simulink model "tcs_VHF_PI_1"  (R2021a)
settings: Solver=FixedStepAuto  StartTime=0.0  StopTime=5  RelTol=1e-3
PreLoadFcn:
  | run('control_bus.m')
model workspace (MAT data in the model file):
  Tmax = 1000
libraries: simulink x2, Solver_SF x1
CloseFcn:
  | clear control_info_bus
settings Model: OrderedModelArguments=off  Creator=henri  LastModifiedBy=Henrique Mesquita

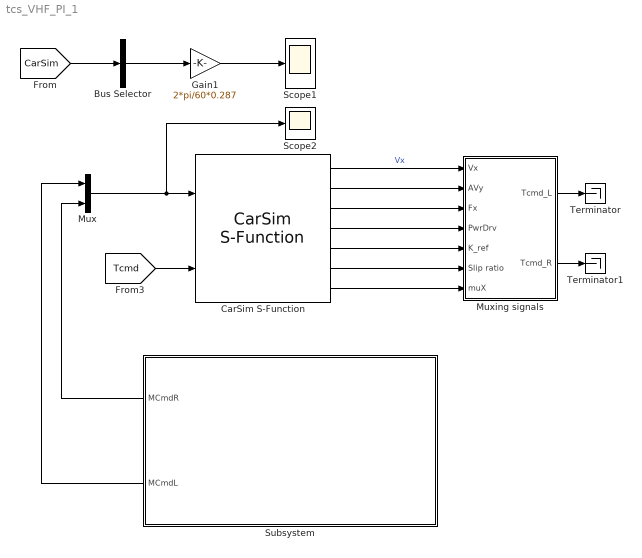
== system tcs_VHF_PI_1 ==
  Bus Selector : BusSelector  OutputSignals=AVy_L1,AVy_R1,AVy_L2,AVy_R2  OutputAsBus=on
  CarSim S-Function : Solver_SF/CarSim S-Function  Priority=1  SIMFILE=simfile.sim  Run_RTs=off  vs_state_ind=Run  StopMode_ind=Vehicle Model
  Gain1 : Gain  Gain=2*pi/60*0.287
  Mux : Mux  Inputs=2
  Muxing signals : Subsystem
  Scope1 : Scope
  Scope2 : Scope
  Subsystem : Subsystem
  Terminator : Terminator
  Terminator1 : Terminator
  wires:
  Mux/1 -> CarSim S-Function/1, Scope2/1
  [CarSim] -> Bus Selector/1
  Bus Selector/1 -> Gain1/1
  Gain1/1 -> Scope1/1
  [Tcmd] -> CarSim S-Function/2
  CarSim S-Function/7 -> Muxing signals/7(muX)
  Muxing signals/2(Tcmd_R) -> Terminator1/1
  CarSim S-Function/6 -> Muxing signals/6(Slip ratio)
  CarSim S-Function/1 -> Muxing signals/1(Vx)  "Vx"
  CarSim S-Function/3 -> Muxing signals/3(Fx)
  CarSim S-Function/2 -> Muxing signals/2(AVy)
  CarSim S-Function/5 -> Muxing signals/5(K_ref)
  CarSim S-Function/4 -> Muxing signals/4(PwrDrv)
  Muxing signals/1(Tcmd_L) -> Terminator/1
  Subsystem/2(MCmdL) -> Mux/1
  Subsystem/1(MCmdR) -> Mux/2

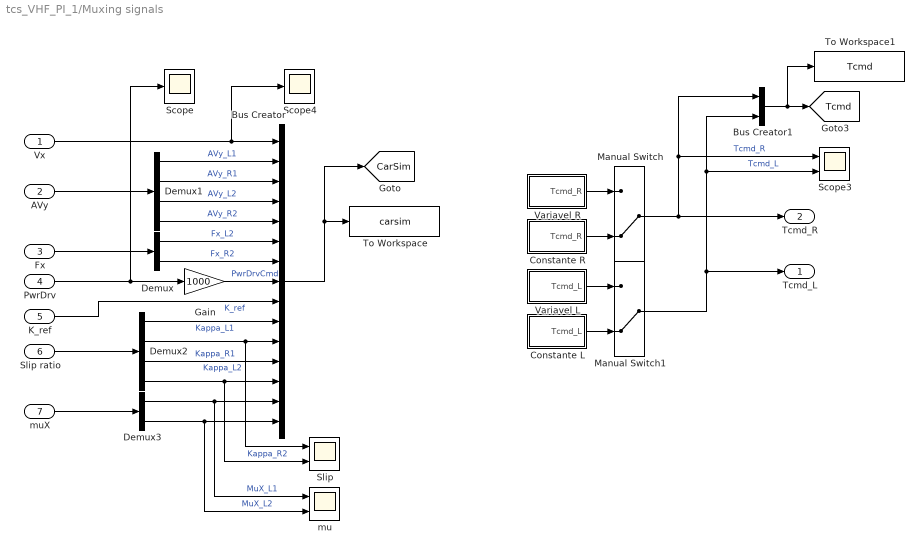
== system tcs_VHF_PI_1/Muxing signals ==
  Vx : Inport
  AVy : Inport  Port=2
  Fx : Inport  Port=3
  PwrDrv : Inport  Port=4
  K_ref : Inport  Port=5
  Slip ratio : Inport  Port=6
  muX : Inport  Port=7
  Bus Creator : BusCreator  Inputs=15
  Bus Creator1 : BusCreator  Inputs=2
  Constante L : Subsystem
  Constante R : Subsystem
  Demux : Demux  Outputs=2
  Demux1 : Demux
  Demux2 : Demux
  Demux3 : Demux  Outputs=2
  Gain : Gain  Gain=1000
  Manual Switch : ManualSwitch  CurrentSetting=0
  Manual Switch1 : ManualSwitch  CurrentSetting=0
  Scope : Scope
  Scope3 : Scope  NumInputPorts=2
  Scope4 : Scope
  Slip : Scope  NumInputPorts=2
  To Workspace : ToWorkspace  VariableName=carsim  SaveFormat=Timeseries  SampleTime=-1
  To Workspace1 : ToWorkspace  VariableName=Tcmd  SaveFormat=Timeseries  SampleTime=-1
  Variavel L : Subsystem
  Variavel R : Subsystem
  mu : Scope  NumInputPorts=2
  Tcmd_L : Outport
  Tcmd_R : Outport  Port=2
  tag scope: CarSim=global, Tcmd=global
  wires:
  K_ref/1 -> Bus Creator/9  "K_ref"
  Demux1/3 -> Bus Creator/4  "AVy_L2"
  Bus Creator/1 -> [CarSim], To Workspace/1
  Demux/2 -> Bus Creator/7  "Fx_R2"
  Vx/1 -> Scope4/1, Bus Creator/1
  Demux1/1 -> Bus Creator/2  "AVy_L1"
  Demux1/4 -> Bus Creator/5  "AVy_R2"
  PwrDrv/1 -> Gain/1, Scope/1
  Demux/1 -> Bus Creator/6  "Fx_L2"
  Gain/1 -> Bus Creator/8  "PwrDrvCmd"
  Demux1/2 -> Bus Creator/3  "AVy_R1"
  Fx/1 -> Demux/1
  AVy/1 -> Demux1/1
  Bus Creator1/1 -> To Workspace1/1, [Tcmd]
  Manual Switch/1 -> Bus Creator1/1, Scope3/1, Tcmd_R/1  "Tcmd_R"
  Manual Switch1/1 -> Bus Creator1/2, Scope3/2, Tcmd_L/1  "Tcmd_L"
  Slip ratio/1 -> Demux2/1
  Demux2/1 -> Bus Creator/10  "Kappa_L1"
  Demux2/2 -> Slip/1, Bus Creator/11  "Kappa_L2"
  Demux2/3 -> Bus Creator/12  "Kappa_R1"
  Demux2/4 -> Slip/2, Bus Creator/13  "Kappa_R2"
  Variavel R/1(Tcmd_R) -> Manual Switch/1
  Constante R/1(Tcmd_R) -> Manual Switch/2
  Constante L/1(Tcmd_L) -> Manual Switch1/2
  Variavel L/1(Tcmd_L) -> Manual Switch1/1
  muX/1 -> Demux3/1
  Demux3/1 -> mu/1, Bus Creator/14  "MuX_L1"
  Demux3/2 -> mu/2, Bus Creator/15  "MuX_L2"

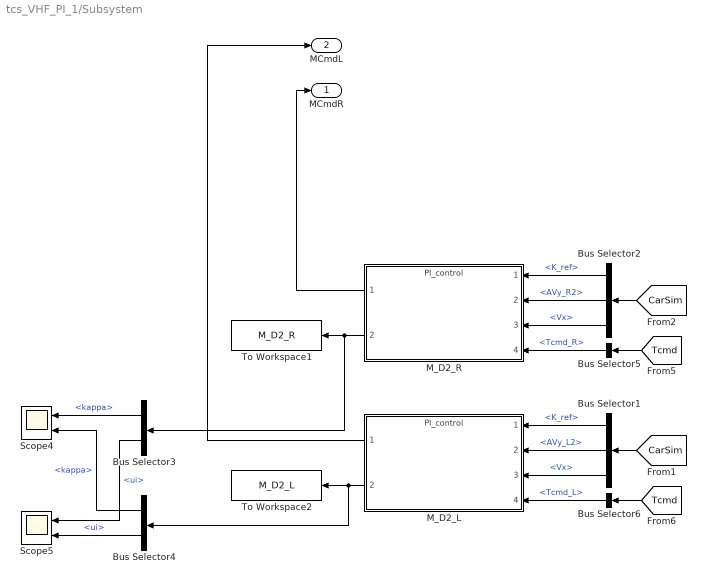
== system tcs_VHF_PI_1/Subsystem ==
  Bus Selector1 : BusSelector  OutputSignals=K_ref,AVy_L2,Vx
  Bus Selector2 : BusSelector  OutputSignals=K_ref,AVy_R2,Vx
  Bus Selector3 : BusSelector  OutputSignals=kappa,ui
  Bus Selector4 : BusSelector  OutputSignals=kappa,ui
  Bus Selector5 : BusSelector  OutputSignals=Tcmd_R
  Bus Selector6 : BusSelector  OutputSignals=Tcmd_L
  M_D2_L : ModelReference  ModelNameDialog=PI_control.slx  SimulationMode=Normal  ModelReferenceVersion=1.23
  M_D2_R : ModelReference  ModelNameDialog=PI_control.slx  SimulationMode=Normal  ModelReferenceVersion=1.23
  Scope4 : Scope  NumInputPorts=2
  Scope5 : Scope  NumInputPorts=2
  To Workspace1 : ToWorkspace  VariableName=M_D2_R  SaveFormat=Timeseries  SampleTime=-1
  To Workspace2 : ToWorkspace  VariableName=M_D2_L  SaveFormat=Timeseries  SampleTime=-1
  MCmdR : Outport
  MCmdL : Outport  Port=2
  wires:
  M_D2_L/2 -> Bus Selector4/1, To Workspace2/1
  M_D2_R/2 -> Bus Selector3/1, To Workspace1/1
  Bus Selector1/2 -> M_D2_L/2  "<AVy_L2>"
  Bus Selector6/1 -> M_D2_L/4  "<Tcmd_L>"
  [Tcmd] -> Bus Selector6/1
  [CarSim] -> Bus Selector2/1
  [Tcmd] -> Bus Selector5/1
  Bus Selector5/1 -> M_D2_R/4  "<Tcmd_R>"
  [CarSim] -> Bus Selector1/1
  Bus Selector1/3 -> M_D2_L/3  "<Vx>"
  Bus Selector2/3 -> M_D2_R/3  "<Vx>"
  Bus Selector4/1 -> Scope4/2  "<kappa>"
  Bus Selector3/2 -> Scope5/1  "<ui>"
  Bus Selector4/2 -> Scope5/2  "<ui>"
  Bus Selector3/1 -> Scope4/1  "<kappa>"
  M_D2_R/1 -> MCmdR/1
  Bus Selector2/2 -> M_D2_R/2  "<AVy_R2>"
  Bus Selector1/1 -> M_D2_L/1  "<K_ref>"
  Bus Selector2/1 -> M_D2_R/1  "<K_ref>"
  M_D2_L/1 -> MCmdL/1

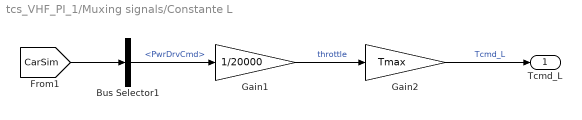
== system tcs_VHF_PI_1/Muxing signals/Constante L ==
  Bus Selector1 : BusSelector  OutputSignals=PwrDrvCmd
  Gain1 : Gain  Gain=1/20000
  Gain2 : Gain  Gain=Tmax
  Tcmd_L : Outport
  wires:
  Gain2/1 -> Tcmd_L/1  "Tcmd_L"
  Gain1/1 -> Gain2/1  "throttle"
  [CarSim] -> Bus Selector1/1
  Bus Selector1/1 -> Gain1/1  "<PwrDrvCmd>"

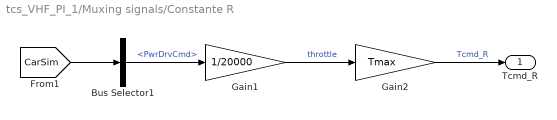
== system tcs_VHF_PI_1/Muxing signals/Constante R ==
  Bus Selector1 : BusSelector  OutputSignals=PwrDrvCmd
  Gain1 : Gain  Gain=1/20000
  Gain2 : Gain  Gain=Tmax
  Tcmd_R : Outport
  wires:
  Gain2/1 -> Tcmd_R/1  "Tcmd_R"
  Gain1/1 -> Gain2/1  "throttle"
  [CarSim] -> Bus Selector1/1
  Bus Selector1/1 -> Gain1/1  "<PwrDrvCmd>"

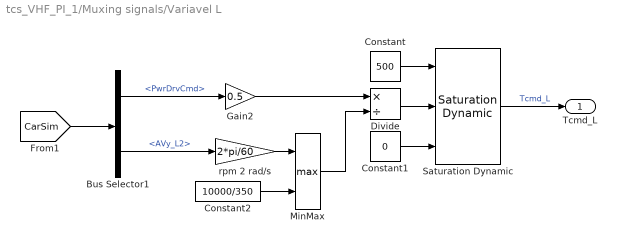
== system tcs_VHF_PI_1/Muxing signals/Variavel L ==
  Bus Selector1 : BusSelector  OutputSignals=PwrDrvCmd,AVy_L2
  Constant : Constant  Value=500
  Constant1 : Constant  Value=0
  Constant2 : Constant  Value=10000/350
  Divide : Product  Inputs=*/
  Gain2 : Gain  Gain=0.5
  MinMax : MinMax  Function=max  Inputs=2
  Saturation Dynamic : simulink/Discontinuities/Saturation Dynamic  OutMin=[]  OutMax=[]  OutDataTypeStr=Inherit: Same as second input  OutDataType=fixdt(1, 16)  OutScaling=2^-10  DoSatur=off
  rpm 2 rad/s : Gain  Gain=2*pi/60
  Tcmd_L : Outport
  wires:
  [CarSim] -> Bus Selector1/1
  Bus Selector1/1 -> Gain2/1  "<PwrDrvCmd>"
  Divide/1 -> Saturation Dynamic/2
  Constant1/1 -> Saturation Dynamic/3
  Bus Selector1/2 -> rpm 2 rad/s/1  "<AVy_L2>"
  Gain2/1 -> Divide/1
  Saturation Dynamic/1 -> Tcmd_L/1  "Tcmd_L"
  rpm 2 rad/s/1 -> MinMax/1
  MinMax/1 -> Divide/2
  Constant2/1 -> MinMax/2
  Constant/1 -> Saturation Dynamic/1

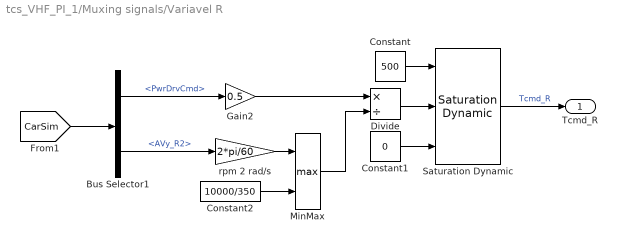
== system tcs_VHF_PI_1/Muxing signals/Variavel R ==
  Bus Selector1 : BusSelector  OutputSignals=PwrDrvCmd,AVy_R2
  Constant : Constant  Value=500
  Constant1 : Constant  Value=0
  Constant2 : Constant  Value=10000/350
  Divide : Product  Inputs=*/
  Gain2 : Gain  Gain=0.5
  MinMax : MinMax  Function=max  Inputs=2
  Saturation Dynamic : simulink/Discontinuities/Saturation Dynamic  OutMin=[]  OutMax=[]  OutDataTypeStr=Inherit: Same as second input  OutDataType=fixdt(1, 16)  OutScaling=2^-10  DoSatur=off
  rpm 2 rad/s : Gain  Gain=2*pi/60
  Tcmd_R : Outport
  wires:
  [CarSim] -> Bus Selector1/1
  Bus Selector1/1 -> Gain2/1  "<PwrDrvCmd>"
  Divide/1 -> Saturation Dynamic/2
  Constant1/1 -> Saturation Dynamic/3
  Bus Selector1/2 -> rpm 2 rad/s/1  "<AVy_R2>"
  Constant/1 -> Saturation Dynamic/1
  Gain2/1 -> Divide/1
  Saturation Dynamic/1 -> Tcmd_R/1  "Tcmd_R"
  rpm 2 rad/s/1 -> MinMax/1
  MinMax/1 -> Divide/2
  Constant2/1 -> MinMax/2
